simulink model "Schemabloc"  (R2016a)
settings: Solver=VariableStepAuto  StartTime=0.0  StopTime=10.0  RelTol=1e-3
undefined symbols (not defined in the file): beq, Jeq, K, L, R, r, rv
libraries: simulink x1
settings Model: Creator=PC  LastModifiedBy=PC

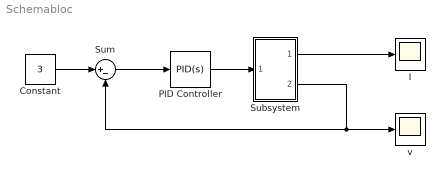
== system Schemabloc ==
  Constant : Constant  Value=3
  I : Scope
  PID Controller : simulink/Continuous/PID Controller  Controller=PID  TimeDomain=Continuous-time  SampleTime=-1  IntegratorMethod=Forward Euler  FilterMethod=Forward Euler  Form=Parallel  UseFilter=on  ControllerParametersSource=internal  P=67.113375324477  I=142.126635801479  D=-0.279755556113956  N=239.900062242692  InitialConditionSource=internal  InitialConditionForIntegrator=0  InitialConditionForFilter=0  ExternalReset=none  LimitOutput=off  UpperSaturationLimit=inf  LowerSaturationLimit=-inf  LinearizeAsGain=on  AntiWindupMode=none  Kb=1  TrackingMode=off  Kt=1  PParamMin=[]  PParamMax=[]  IParamMin=[]  IParamMax=[]  DParamMin=[]  DParamMax=[]  NParamMin=[]  NParamMax=[]  KbParamMin=[]  KbParamMax=[]  KtParamMin=[]  KtParamMax=[]  POutMin=[]  POutMax=[]  IOutMin=[]  IOutMax=[]  DOutMin=[]  DOutMax=[]  NOutMin=[]  NOutMax=[]  KbOutMin=[]  KbOutMax=[]  KtOutMin=[]  KtOutMax=[]  IntegratorOutMin=[]  IntegratorOutMax=[]  FilterOutMin=[]  FilterOutMax=[]  SumOutMin=[]  SumOutMax=[]  SumI1OutMin=[]  SumI1OutMax=[]  SumI2OutMin=[]  SumI2OutMax=[]  SumI3OutMin=[]  SumI3OutMax=[]  SumDOutMin=[]  SumDOutMax=[]  SaturationOutMin=[]  SaturationOutMax=[]  IntegratorContinuousStateAttributes=''  IntegratorStateMustResolveToSignalObject=off  IntegratorRTWStateStorageClass=Auto  FilterContinuousStateAttributes=''  FilterStateMustResolveToSignalObject=off  FilterRTWStateStorageClass=Auto  DifferentiatorICPrevScaledInput=0  DifferentiatorOutMin=[]  DifferentiatorOutMax=[]
  Subsystem : Subsystem
  Sum : Sum  Inputs=|+-
  v : Scope
  wires:
  Subsystem/1(Out1) -> I/1
  Subsystem/2(Out2) -> v/1, Sum/2
  PID Controller/1 -> Subsystem/1(In1)
  Sum/1 -> PID Controller/1
  Constant/1 -> Sum/1

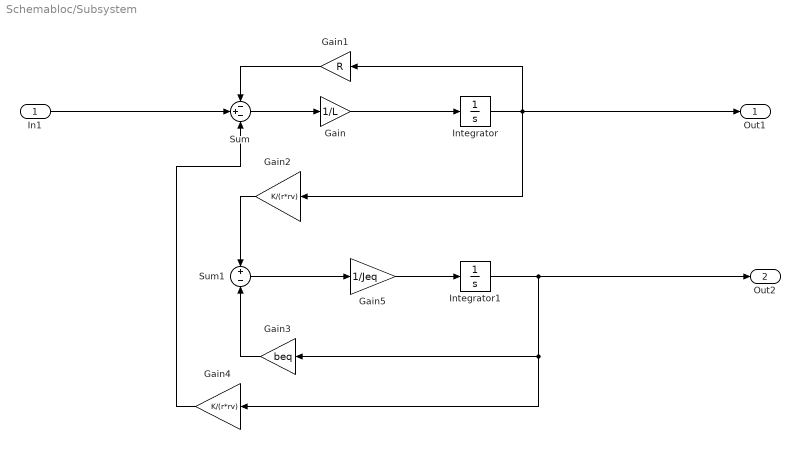
== system Schemabloc/Subsystem ==
  In1 : Inport
  Gain : Gain  Gain=1/L
  Gain1 : Gain  Gain=R
  Gain2 : Gain  Gain=K/(r*rv)
  Gain3 : Gain  Gain=beq
  Gain4 : Gain  Gain=K/(r*rv)
  Gain5 : Gain  Gain=1/Jeq
  Integrator : Integrator
  Integrator1 : Integrator
  Sum : Sum  Inputs=-+-
  Sum1 : Sum  Inputs=+-
  Out1 : Outport
  Out2 : Outport  Port=2
  wires:
  Integrator/1 -> Out1/1, Gain2/1, Gain1/1
  Integrator1/1 -> Out2/1, Gain3/1, Gain4/1
  Gain5/1 -> Integrator1/1
  Sum1/1 -> Gain5/1
  In1/1 -> Sum/2
  Gain4/1 -> Sum/3
  Gain1/1 -> Sum/1
  Gain/1 -> Integrator/1
  Sum/1 -> Gain/1
  Gain3/1 -> Sum1/2
  Gain2/1 -> Sum1/1
